simulink model "plant_model_testing"  (R2021a)
settings: Solver=VariableStepAuto  StartTime=0.0  StopTime=10.0  RelTol=1e-3
undefined symbols (not defined in the file): sigbuilder_block
settings Model: Creator=46769  LastModifiedBy=46769

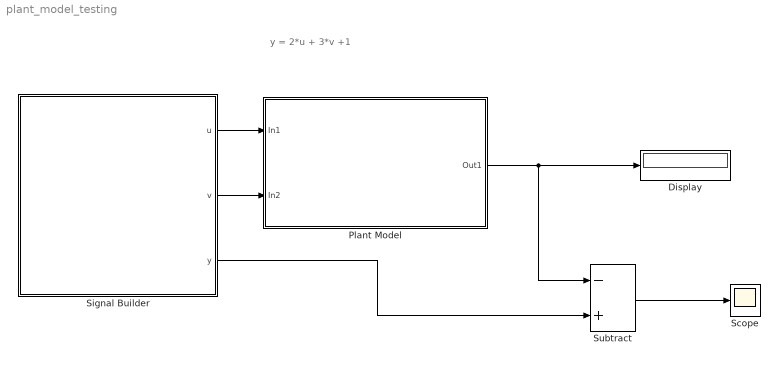
== system plant_model_testing ==
  note: y = 2*u + 3*v +1
  Display : Display
  Plant Model : Subsystem
  Scope : Scope
  Signal Builder : Subsystem  Tag=STV Subsys  LoadFcn=sigbuilder_block('load');  StartFcn=sigbuilder_block('start');  StopFcn=sigbuilder_block('stop');  ClipboardFcn=sigbuilder_block('clipboard');  mask(Sigbuilder block){tuvar=[0:10]}
      mask help: Simulink:masks:SigbuilderBlock_MD
      mask init:
      | if ~strcmp(get_param(bdroot(gcbh),'SimulationStatus'),'stopped') tuvar = sigbuilder_block('maskInit'); end
      settings: CopyFcn=sigbuilder_block('copy');  DeleteFcn=sigbuilder_block('delete');  ModelCloseFcn=sigbuilder_block('modelClose');  PreSaveFcn=sigbuilder_block('preSave');  PauseFcn=sigbuilder_block('pause');  ContinueFcn=sigbuilder_block('continue');  NameChangeFcn=sigbuilder_block('namechange');  OpenFcn=sigbuilder_block('open',[494.4 102.6 550.8 400.2 ]);  CloseFcn=sigbuilder_block('close');
      mask Display: plot(0, 0, 100, 100,[2, 2, 32, 32, 2], [68, 8, 8, 68, 68],[32, 2], [38, 38], [32, 19, 2],[53, 60, 44], [32, 17, 17, 2],[16, 16, 31, 31]);txt = getActiveGroup(gcbh);text(2, 100, txt,'verticalAlignment', 'top');
  Subtract : Sum  Inputs=-+
  wires:
  Plant Model/1(Out1) -> Subtract/1, Display/1
  Signal Builder/1(u) -> Plant Model/1(In1)
  Signal Builder/2(v) -> Plant Model/2(In2)
  Signal Builder/3(y) -> Subtract/2
  Subtract/1 -> Scope/1

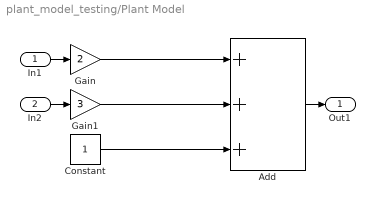
== system plant_model_testing/Plant Model ==
  In1 : Inport
  In2 : Inport  Port=2
  Add : Sum  Inputs=+++
  Constant : Constant
  Gain : Gain  Gain=2
  Gain1 : Gain  Gain=3
  Out1 : Outport
  wires:
  Constant/1 -> Add/3
  Gain1/1 -> Add/2
  In2/1 -> Gain1/1
  In1/1 -> Gain/1
  Add/1 -> Out1/1
  Gain/1 -> Add/1

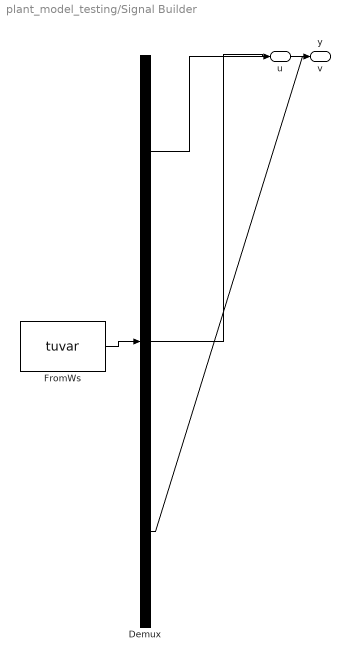
== system plant_model_testing/Signal Builder ==
  Demux : Demux  Tag=STV Demux  Outputs=3
      settings: DisplayOption=none
  FromWs : FromWorkspace  Tag=STV FromWs  VariableName=tuvar
      SigBuilderData=|
      | common.afterFinalStr = 'Extrapolate'
      | common.sampleTime = 0
      | dataSet.timeRange = [0 10]
      | dataSet.name = 'Group 1'
      | sbobj.Groups.Name = 'Group 1'
      | sbobj.Groups.Signals(1).Name = 'u'
      | sbobj.Groups.Signals(1).XData = [0 2 2 6 6 10]
      | sbobj.Groups.Signals(1).YData = [0 0 2 2 0 0]
      | sbobj.Groups.Signals(2).Name = 'v'
      | sbobj.Groups.Signals(2).XData = [0 4 4 9 9 10]
      | sbobj.Groups.Signals(2).YData = [0 0 3 3 0 0]
      | sbobj.Groups.Signals(3).Name = 'y'
      | sbobj.Groups.Signals(3).XData = [0 2 2 4 4 6 6 9 9 10]
      | sbobj.Groups.Signals(3).YData = [1 1 5 5 14 14 10 10 1 1]
  u : Outport  Tag=STV Outport
  v : Outport  Tag=STV Outport  Port=2
  y : Outport  Tag=STV Outport  Port=3
  wires:
  Demux/1 -> u/1
  FromWs/1 -> Demux/1
  Demux/2 -> v/1
  Demux/3 -> y/1
